simulink model "BallAndBeamTest"  (R2019a)
settings: Solver=ode4  StartTime=0.0  StopTime=inf  FixedStep=0.002  RelTol=1e-3
undefined symbols (not defined in the file): HIL, qc_get_step_size
libraries: quarc_library x5, simulink x1
settings Model: ExtModeTrigDuration=5000  Creator=Rchan  LastModifiedBy=pmartin
settings DebuggingCC: UnderspecifiedInitializationDetection=Classic  MergeDetectMultiDrivingBlocksExec=none
settings ModelReferenceCC: PropagateSignalLabelsOutOfModel=off

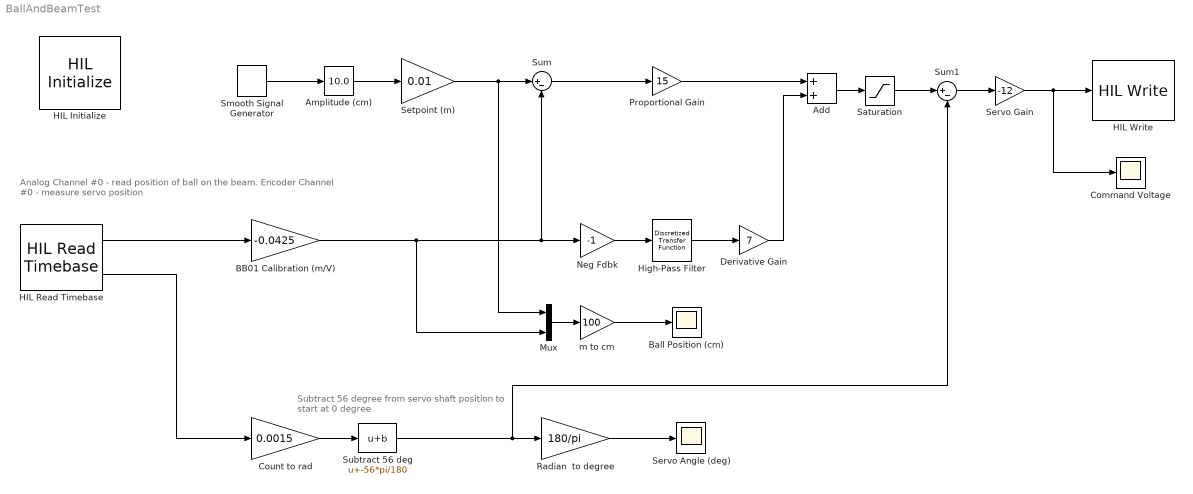
== system BallAndBeamTest ==
  note: Analog Channel #0 - read position of ball on the beam.
      | Encoder Channel #0 - measure servo position
  note: Subtract 56 degree from servo shaft
      | position to start at 0 degree
  Add : Sum
  Amplitude (cm) : simulink/Math Operations/Slider Gain  gain=10.0  low=-10  high=10
  BB01 Calibration (m/V) : Gain  Gain=-0.0425  SaturateOnIntegerOverflow=on  OutDataTypeStr=Inherit: Same as input  ParamDataTypeStr=Inherit: Same as input
  Ball Position (cm) : Scope
  Command Voltage : Scope
  Count to rad : Gain  Gain=0.0015  SaturateOnIntegerOverflow=on  OutDataTypeStr=Inherit: Same as input  ParamDataTypeStr=Inherit: Same as input
  Derivative Gain : Gain  Gain=7
  HIL Initialize : quarc_library/Data Acquisition/Generic/Configuration/HIL Initialize  object_name=HIL-1  board_type=q8_usb  board_number=0@tcpip://localhost:18942  board_options=update_rate=normal  exclusive=off  active=on  hardware_clocks=[0:2]  clock_modes=[]  initial_clock_frequencies=[]  set_clock_params_at_start=off  set_clock_params_at_switch_in=off  set_clock_frequencies_at_start=off  set_clock_frequencies_at_switch_in=off  analog_input_channels=[0:7]  analog_input_configurations=[]  analog_input_maximums=10  analog_input_minimums=-10  set_analog_input_params_at_start=on  set_analog_input_params_at_switch_in=off  analog_output_channels=[0:7]  analog_output_maximums=10  analog_output_minimums=-10  initial_analog_outputs=[0]  final_analog_outputs=[0]  watchdog_analog_outputs=0  set_analog_output_params_at_start=on  set_analog_output_params_at_switch_in=off  set_analog_outputs_at_start=on  set_analog_outputs_at_switch_in=off  set_analog_outputs_at_terminate=on  set_analog_outputs_at_switch_out=off  set_analog_outputs_on_watchdog=off  digital_input_channels=[]  digital_output_channels=[0:7]  digital_output_configuration=[]  initial_digital_outputs=[0]  final_digital_outputs=[0]  watchdog_digital_outputs=[0]  set_digital_output_params_at_start=off  set_digital_output_params_at_switch_in=off  set_digital_outputs_at_start=on  set_digital_outputs_at_switch_in=off  set_digital_outputs_at_terminate=on  set_digital_outputs_at_switch_out=off  set_digital_outputs_on_watchdog=off  encoder_channels=[0:7]  quadrature=[4]  encoder_filter_frequency=[]  initial_encoder_counts=[0]  set_encoder_params_at_start=on  set_encoder_params_at_switch_in=off  set_encoder_counts_at_start=on  set_encoder_counts_at_switch_in=off  pwm_channels=[0:7]  pwm_modes=0  pwm_frequency=99.532799999999995e6/4095  pwm_configuration=[0]  pwm_alignment=[0]  pwm_polarity=[1]  pwm_leading_deadband=[0]  pwm_trailing_deadband=[0]  initial_pwm_outputs=[0]  final_pwm_outputs=[0]  watchdog_pwm_outputs=[0]  set_pwm_params_at_start=on  set_pwm_params_at_switch_in=off  set_pwm_outputs_at_start=on  set_pwm_outputs_at_switch_in=off  set_pwm_outputs_at_terminate=on  set_pwm_outputs_at_switch_out=off  set_pwm_outputs_on_watchdog=off  other_output_channels=[]  initial_other_outputs=[]  final_other_outputs=[]  watchdog_other_outputs=[]  set_other_outputs_at_start=off  set_other_outputs_at_switch_in=off  set_other_outputs_at_terminate=off  set_other_outputs_at_switch_out=off  set_other_outputs_on_watchdog=off
  HIL Read Timebase : quarc_library/Data Acquisition/Generic/Timebases/HIL Read Timebase  object_name=HIL-1  clock=0  analog_channels=[0]  encoder_channels=[0]  digital_channels=[]  other_channels=[]  active=on  vector_output=off  data_type_mode=Inherit via back propagation  encoder_data_type=double  digital_data_type=boolean  overflow_mode=Synchronize (for simulated cards only)  samples_in_buffer=1+0*max(ceil(1/qc_get_step_size), 1)
  HIL Write : quarc_library/Data Acquisition/Generic/Immediate I//O/HIL Write  object_name=HIL-1  analog_channels=0  pwm_channels=[]  digital_channels=[]  other_channels=[]  sample_time=-1  active=on  vector_input=off
  High-Pass Filter : quarc_library/Discrete/Discretized Transfer Function  num=[15 0]  den=[1 15]  method=tustin  Ts=qc_get_step_size
      settings: SourceProductName=QUARC Targets
  Mux : Mux  Inputs=2
  Neg Fdbk : Gain  Gain=-1  SaturateOnIntegerOverflow=on  OutDataTypeStr=Inherit: Same as input  ParamDataTypeStr=Inherit: Same as input
  Proportional Gain : Gain  Gain=15
  "Radian  to degree " : Gain  Gain=180/pi  SaturateOnIntegerOverflow=on  OutDataTypeStr=Inherit: Same as input  ParamDataTypeStr=Inherit: Same as input
  Saturation : Saturate  UpperLimit=0.9774  LowerLimit=-0.9774
  Servo Angle (deg) : Scope
  Servo Gain : Gain  Gain=-12
  Setpoint (m) : Gain  Gain=0.01
  Smooth Signal Generator : quarc_library/Sources/Signals/Smooth Signal Generator  signal_type=Square  source=Internal (dialog parameters)  amplitude=1  frequency=0.08  initial_phase=0  sample_time=qc_get_step_size  output_cos=off
      settings: SourceProductName=QUARC Targets
  Subtract 56 deg : Bias  Bias=-56*pi/180
  Sum : Sum  Inputs=|+-
  Sum1 : Sum  Inputs=|+-
  m to cm : Gain  Gain=100  SaturateOnIntegerOverflow=on  OutDataTypeStr=Inherit: Same as input  ParamDataTypeStr=Inherit: Same as input
  wires:
  Smooth Signal Generator/1 -> Amplitude (cm)/1
  Amplitude (cm)/1 -> Setpoint (m)/1
  Sum/1 -> Proportional Gain/1
  HIL Read Timebase/1 -> BB01 Calibration (m/V)/1
  Setpoint (m)/1 -> Sum/1, Mux/1
  BB01 Calibration (m/V)/1 -> Sum/2, Neg Fdbk/1, Mux/2
  "Radian  to degree "/1 -> Servo Angle (deg)/1
  Neg Fdbk/1 -> High-Pass Filter/1
  High-Pass Filter/1 -> Derivative Gain/1
  Proportional Gain/1 -> Add/1
  Derivative Gain/1 -> Add/2
  Servo Gain/1 -> HIL Write/1, Command Voltage/1
  Add/1 -> Saturation/1
  Sum1/1 -> Servo Gain/1
  m to cm/1 -> Ball Position (cm)/1
  Saturation/1 -> Sum1/1
  Count to rad/1 -> Subtract 56 deg/1
  Subtract 56 deg/1 -> "Radian  to degree "/1, Sum1/2
  Mux/1 -> m to cm/1
  HIL Read Timebase/2 -> Count to rad/1
